simulink library "lib_transmission2"  (Simulink 4.1.1)
values from neighbouring files (symbols this model uses):
  logFlag = 1    [advSACompMaskInit.m]    (also in advSACompMaskInitR13.m)
undefined symbols (not defined in the file or in its folder): cyc_mph, fc_map_spd, fc_max_trq, fc_spd_scale, fc_trq_scale, fd_inertia, fd_loss, fd_ratio, gb_dnshift_load, gb_dnshift_spd, gb_gear_number_lookup, gb_gears_num, gb_inertia, gb_loss_const, gb_loss_input_spd_coeff, gb_loss_input_trq_coeff, gb_loss_output_spd_coeff, gb_loss_output_trq_coeff, gb_map_spd_out, gb_map_trq_in, gb_map_trq_out, gb_num_init, gb_ratio, gb_shift_delay, gb_spd_scale, gb_trq_scale, gb_upshift_load, gb_upshift_spd, htc_inertia, htc_k_adv, htc_k_adv_coast, htc_lockup, htc_lockup_load, htc_lockup_spd, htc_lu_gear_range, htc_max_coast_tr, htc_min_coast_tr, htc_pump_loss_spd, htc_pump_loss_trq_lockup, htc_pump_loss_trq_unlock, htc_sr, htc_sr_coast, htc_tr, htc_tr_coast, htc_unlock_spd, mc_map_spd, mc_max_trq, mc_overtrq_factor, mc_spd_scale, mc_trq_scale, tc_loss, tc_mc_to_fc_ratio, tx_eff_map, tx_map_spd, tx_map_trq, tx_pg_r, tx_pg_s, tx_speed_dep, vc_clutch_bool, vc_idle_spd ... (+2)
libraries: lib_controls x1, lib_etc x1, lib_controls2 x1, lib_transmission x1
(part 2 of 17)

== system lib_transmission2/SubLibraries/loss (Nm) old methodology ==
  note: Loss torque applied at input side is a function of
      |  output speed, output torque, and gear number.
      | There is no loss if the gears are not turning.
  "output torque and speed (Nm), (rad/s)" : Inport  Port=1  LatchInput=off
  gear ratio : Inport  Port=2  LatchInput=off
  Abs : Abs  SaturateOnIntegerOverflow=on
  Block NOTES : Subsystem
      settings: RTWFcnNameOpts=Auto  RTWFileNameOpts=Auto
      mask Display: disp('Block\nNOTES')
  Constant : Constant  Orientation=up  Value=eps
  Constant1 : Constant  Value=gb_loss_input_spd_coeff/gb_spd_scale
  Constant2 : Constant  Value=gb_loss_input_trq_coeff/gb_trq_scale
  Constant3 : Constant  Value=gb_loss_output_spd_coeff/gb_spd_scale
  Constant4 : Constant  Value=gb_loss_output_trq_coeff/gb_trq_scale
  Constant5 : Constant  Orientation=up  Value=gb_loss_const
  Constant6 : Constant  Value=gb_loss_output_pwr_coeff/gb_spd_scale/gb_trq_scale
  Constant7 : Constant  Orientation=up  Value=0
  Demux : Demux  Outputs=2  BusSelectionMode=off
  Product : Product  Inputs=2  Multiplication=Element-wise(.*)  SaturateOnIntegerOverflow=on
  Product1 : Product  Inputs=/*  Multiplication=Element-wise(.*)  SaturateOnIntegerOverflow=on
  Product2 : Product  Inputs=2  Multiplication=Element-wise(.*)  SaturateOnIntegerOverflow=on
  Product3 : Product  Inputs=2  Multiplication=Element-wise(.*)  SaturateOnIntegerOverflow=on
  Product4 : Product  Inputs=3  Multiplication=Element-wise(.*)  SaturateOnIntegerOverflow=on
  Relational Operator : RelationalOperator  Operator=>
  Saturation : Saturate  UpperLimit=inf  LowerLimit=0  LinearizeAsGain=on
  Sum : Sum  Inputs=++  SaturateOnIntegerOverflow=on
  Sum1 : Sum  Inputs=++  SaturateOnIntegerOverflow=on
  Sum2 : Sum  Inputs=++++  SaturateOnIntegerOverflow=on
  Sum3 : Sum  Orientation=up  Inputs=++  SaturateOnIntegerOverflow=on
  Switch : Switch  Threshold=eps
  loss torque : Product  Inputs=*//  Multiplication=Element-wise(.*)  SaturateOnIntegerOverflow=on
  loss torque at input shaft (Nm) : Outport  Port=1  InitialOutput=0
  wires:
  Abs/1 -> Product2/1, Product4/1
  Demux/1 -> Abs/1
  Relational Operator/1 -> Switch/2
  Constant/1 -> Relational Operator/2, Sum3/2
  Constant7/1 -> Switch/3
  Product3/1 -> Sum2/3
  Product2/1 -> Sum2/1
  "output torque and speed (Nm), (rad/s)"/1 -> Demux/1
  Constant1/1 -> Product/2
  Product/1 -> Sum1/2
  Sum/1 -> Product2/2
  Sum1/1 -> Product3/2
  Constant5/1 -> Sum2/4
  gear ratio/1 -> Product1/1, Product/1, loss torque/3
  Constant2/1 -> Product1/2
  Product1/1 -> Sum/2
  Constant4/1 -> Sum/1
  Constant3/1 -> Sum1/1
  Constant6/1 -> Product4/2
  Product4/1 -> Sum2/2
  Switch/1 -> loss torque at input shaft (Nm)/1
  Sum2/1 -> loss torque/1
  Demux/2 -> Product3/1, Product4/3, Relational Operator/1, Sum3/1
  loss torque/1 -> Saturation/1
  Saturation/1 -> Switch/1
  Sum3/1 -> loss torque/2

== system lib_transmission2/SubLibraries/notes on  3D discrete lookup table ==
  note: performs a "2D" lookup
      | for the specified
      | z height of the 3D lookup matrix
      | (i.e., no interpolation on z, only discrete)
  note: created 5 July 2001 mpo
      | Revision history:
      | ...
  note: 3 inputs:
      | (1) X lookup
      | (2) Y lookup
      | (3) discrete Z value (integer)
      |
      | 1 output:
      | (1) looked up value
  note: 3 masked inputs:
      | (1) array of X values in table
      | (2) array of Y values in table
      | (3) 3D lookup table (i.e., 2D tables for several Z values)

== system lib_transmission2/SubLibraries/notes on  loss (Nm) ==
  note: 4 masked inputs:
      | (1) map of efficiencies by spd and trq and gear number (discrete)
      | (2) array of trq values in efficiency map lookup table
      | (3) array of spd values in efficiency map lookup table
      | (4) the ratios in the gear box
  note: 2 inputs:
      | (1) trq and spd at output (wheel side)
      | of Transmission (muxxed)
      | (2) current gear ratio
      |
      | 1 output:
      | (1) trq loss at input (engine side) of
      | transmission
  note: created 5 July 2001 mpo
      | Revision history:
      | ...
  note: Calculates the torque loss due to
      | transmission inefficiencies
      | (torque lost at input to transmission)
  note: note: tx_map_spd and tx_map_trq
      |  are output (wheelside) values
  note: data needs:
      | tx_map_spd
      | tx_map_trq
      | tx_eff_map
      | gb_ratio

== system lib_transmission2/clutch <cl>/clutch model and interface ==
  note: Interface
  note: Model
  T & w output requested : Inport  Port=1  LatchInput=off
  T & w input achieved : Inport  Port=2  LatchInput=off
  control : Inport  Port=3  LatchInput=off
  Bus Creator : BusCreator  Inputs=2
  Demux2 : Demux  Outputs=3  BusSelectionMode=off
  Goto Tag Visibility : GotoTagVisibility  GotoTag=clutch_state
  Goto Tag Visibility1 : GotoTagVisibility  GotoTag=T_cl_out
  Goto Tag Visibility2 : GotoTagVisibility  GotoTag=w_cl_out
  Goto Tag Visibility3 : GotoTagVisibility  GotoTag=launch_speed
  Goto Tag Visibility4 : GotoTagVisibility  GotoTag=launch_flag
  clutch model : Subsystem
      settings: RTWFcnNameOpts=Auto  RTWFileNameOpts=Auto
  signal annotator : Subsystem
      settings: RTWFcnNameOpts=Auto  RTWFileNameOpts=Auto
  required out : Outport  Port=1
  Out1 : Outport  Port=2
  Out2 : Outport  Port=3
  sensors : Outport  Port=4
  tag scope: clutch_state=scoped, launch_flag=scoped, launch_speed=scoped
  wires:
  control/1 -> Demux2/1
  Demux2/1 -> [clutch_state]
  Demux2/2 -> [launch_speed]
  Demux2/3 -> [launch_flag]
  [T_cl_out] -> Bus Creator/1  "T_cl_out"
  [w_cl_out] -> Bus Creator/2  "w_cl_out"
  T & w output requested/1 -> clutch model/1(T & w output requested), signal annotator/1(In1)
  clutch model/1(T & w input request) -> Out1/1
  T & w input achieved/1 -> clutch model/2(T & w input achieved)
  clutch model/2(T & w output achieved) -> Out2/1
  Bus Creator/1 -> sensors/1
  signal annotator/1(Out1) -> required out/1

== system lib_transmission2/final drive <fd>/Block NOTES ==
  note: This final drive model includes loss data, rotational inertia, and a gear reduction.
  note: The loss torque is zero when the gears are not turning,
      | and is applied at the input side of the gear reduction.
  note: The inertia torque is the input torque required to accelerate the
      | final drive's inertia as measured on the input side.

== system lib_transmission2/final drive <fd>/help ==

== system lib_transmission2/final drive <fd>/model&interface ==
  note: Interface
  note: Model
  T & w output request : Inport  Port=1  LatchInput=off
  T & w input achieved : Inport  Port=2  LatchInput=off
  control : Inport  Port=3  LatchInput=off
  Ground : Ground
  Terminator : Terminator
  model : Subsystem
      settings: RTWFcnNameOpts=Auto  RTWFileNameOpts=Auto
  signal annotator : Subsystem
      settings: RTWFcnNameOpts=Auto  RTWFileNameOpts=Auto
  out request : Outport  Port=1  InitialOutput=0
  T & w input request : Outport  Port=2  InitialOutput=0
  T & w output achieved : Outport  Port=3  InitialOutput=0
  sensors : Outport  Port=4  InitialOutput=0
  wires:
  model/1("torque and speed req'd at input side of final drive (Nm), (rad/s)") -> T & w input request/1
  T & w output request/1 -> model/1("torque and speed req'd at output side of final drive (Nm), (rad/s)"), signal annotator/1(In1)
  T & w input achieved/1 -> model/2("torque and speed avail. at input side of final drive (Nm), (rad/s)")
  model/2("torque and speed avail. at output side of final drive (Nm), (rad/s)") -> T & w output achieved/1
  Ground/1 -> sensors/1
  control/1 -> Terminator/1
  signal annotator/1(Out1) -> out request/1

== system lib_transmission2/gearbox <gb>/Block NOTES ==
  note: This gearbox model includes loss data, rotational inertia, and a gear reduction.
  note: The loss torque is zero when the gears are not turning,
      | and is applied at the input side of the gear reduction.
  note: The inertia torque is the input torque required to accelerate the
      | final drive's inertia as measured on the input side.
  note: Available output torque is estimated assuming that the gearbox efficiency for theavailable input
      | torque andspeed is the same as the gearbox efficiency for the REQUESTED input torque.
  note: This is a good assumption, at least for the VW 4-speed manual transaxle of SAE 820741.
      | In the VW transaxle, efficiency is fairly independent of torque and speed at high torques.

== system lib_transmission2/gearbox <gb>/gearbox model & interface ==
  note: Model
  note: Interface
  trq and spd output request : Inport  Port=1  LatchInput=off
  trq and spd input achieved : Inport  Port=2  LatchInput=off
  controls : Inport  Port=3  LatchInput=off
  Bus Creator : BusCreator  Inputs=6
  Demux2 : Demux  Outputs=3  BusSelectionMode=off
  Goto Tag Visibility : GotoTagVisibility  GotoTag=gear_number
  Goto Tag Visibility1 : GotoTagVisibility  GotoTag=gb_spd_in_a
  Goto Tag Visibility2 : GotoTagVisibility  GotoTag=gear_ratio
  Goto Tag Visibility3 : GotoTagVisibility  GotoTag=shifting
  Goto Tag Visibility4 : GotoTagVisibility  GotoTag=T_gb_out
  Goto Tag Visibility5 : GotoTagVisibility  GotoTag=w_gb_out
  Goto Tag Visibility6 : GotoTagVisibility  GotoTag=eta_gb
  Goto Tag Visibility7 : GotoTagVisibility  GotoTag=gb_trq_out_a
  Goto Tag Visibility8 : GotoTagVisibility  GotoTag=gb_spd_out_a
  gearbox model : Subsystem
      settings: RTWFcnNameOpts=Auto  RTWFileNameOpts=Auto
  signal annotator : Subsystem
      settings: RTWFcnNameOpts=Auto  RTWFileNameOpts=Auto
  requested output : Outport  Port=1
  trq and spd input request : Outport  Port=2
  trq and spd output achieved : Outport  Port=3
  sensors : Outport  Port=4
  tag scope: gear_number=scoped, gear_ratio=scoped, shifting=scoped
  wires:
  [gb_spd_out_a] -> Bus Creator/6  "gb_spd_out_a"
  [gb_spd_in_a] -> Bus Creator/1  "gb_spd_in_a"
  [T_gb_out] -> Bus Creator/2  "T_gb_out"
  [w_gb_out] -> Bus Creator/3  "w_gb_out"
  [eta_gb] -> Bus Creator/4  "eta_gb"
  Bus Creator/1 -> sensors/1
  controls/1 -> Demux2/1
  Demux2/1 -> [gear_ratio]
  Demux2/2 -> [shifting]
  Demux2/3 -> [gear_number]
  trq and spd output request/1 -> gearbox model/1("torque and speed req'd at output side of gearbox (Nm), (rad/s)"), signal annotator/1(In1)
  gearbox model/1("torque and speed req'd at input side of gearbox (Nm), (rad/s)") -> trq and spd input request/1
  trq and spd input achieved/1 -> gearbox model/2("torque and speed avail. at input side of gearbox (Nm), (rad/s)")
  gearbox model/2("torque and speed avail. at output side of gearbox (Nm), (rad/s)") -> trq and spd output achieved/1
  signal annotator/1(Out1) -> requested output/1
  [gb_trq_out_a] -> Bus Creator/5  "gb_trq_out_a"

== system lib_transmission2/gearbox <gb>/help ==

== system lib_transmission2/gearbox <gb> CVT/Block NOTES ==
  note: This gearbox model includes loss data, rotational inertia, and a gear reduction.
  note: The loss torque is zero when the gears are not turning,
      | and is applied at the input side of the gear reduction.
  note: The inertia torque is the input torque required to accelerate the
      | final drive's inertia as measured on the input side.
  note: Available output torque is estimated assuming that the gearbox efficiency for theavailable input
      | torque andspeed is the same as the gearbox efficiency for the REQUESTED input torque.
  note: This is a good assumption, at least for the VW 4-speed manual transaxle of SAE 820741.
      | In the VW transaxle, efficiency is fairly independent of torque and speed at high torques.

== system lib_transmission2/gearbox <gb> CVT/CVT model & interface ==
  note: Model
  note: Interface
  trq and spd output request : Inport  Port=1  LatchInput=off
  trq and spd input achieved : Inport  Port=2  LatchInput=off
  controls : Inport  Port=3  LatchInput=off
  Bus Creator : BusCreator  Inputs=3
  CVT gearbox  <gb> : Subsystem
      settings: RTWFcnNameOpts=Auto  RTWFileNameOpts=Auto
  Demux2 : Demux  Outputs=1  BusSelectionMode=off
  Goto Tag Visibility2 : GotoTagVisibility  GotoTag=gear_ratio
  Goto Tag Visibility4 : GotoTagVisibility  GotoTag=T_gb_out
  Goto Tag Visibility5 : GotoTagVisibility  GotoTag=w_gb_out
  Goto Tag Visibility6 : GotoTagVisibility  GotoTag=eta_gb
  signal annotator : Subsystem
      settings: RTWFcnNameOpts=Auto  RTWFileNameOpts=Auto
  requested output : Outport  Port=1
  trq and spd input request : Outport  Port=2
  trq and spd output achieved : Outport  Port=3
  sensors : Outport  Port=4
  tag scope: gear_ratio=scoped
  wires:
  Bus Creator/1 -> sensors/1
  controls/1 -> Demux2/1
  Demux2/1 -> [gear_ratio]
  trq and spd output request/1 -> signal annotator/1(In1), CVT gearbox  <gb>/1("torque and speed req'd at output side of cvt (Nm), (rad/s)")
  CVT gearbox  <gb>/1("torque and speed req'd at input side of cvt (Nm), (rad/s)") -> trq and spd input request/1
  trq and spd input achieved/1 -> CVT gearbox  <gb>/2("torque and speed avail. at input side of cvt (Nm), (rad/s)")
  CVT gearbox  <gb>/2("torque and speed avail. at output side of cvt (Nm), (rad/s)") -> trq and spd output achieved/1
  signal annotator/1(Out1) -> requested output/1
  [T_gb_out] -> Bus Creator/1  "T_gb_out"
  [w_gb_out] -> Bus Creator/2  "w_gb_out"
  [eta_gb] -> Bus Creator/3  "eta_gb"

== system lib_transmission2/gearbox <gb> CVT/help ==

== system lib_transmission2/gearbox <gb> old/Block NOTES ==
  note: This gearbox model includes loss data, rotational inertia, and a gear reduction.
  note: The loss torque is zero when the gears are not turning,
      | and is applied at the input side of the gear reduction.
  note: The inertia torque is the input torque required to accelerate the
      | final drive's inertia as measured on the input side.
  note: Available output torque is estimated assuming that the gearbox efficiency for theavailable input
      | torque andspeed is the same as the gearbox efficiency for the REQUESTED input torque.
  note: This is a good assumption, at least for the VW 4-speed manual transaxle of SAE 820741.
      | In the VW transaxle, efficiency is fairly independent of torque and speed at high torques.

== system lib_transmission2/gearbox <gb> old/gearbox model & interface ==
  note: Model
  note: Interface
  trq and spd output request : Inport  Port=1  LatchInput=off
  trq and spd input achieved : Inport  Port=2  LatchInput=off
  controls : Inport  Port=3  LatchInput=off
  Bus Creator : BusCreator  Inputs=5
  Demux2 : Demux  Outputs=3  BusSelectionMode=off
  Goto Tag Visibility : GotoTagVisibility  GotoTag=gear_number
  Goto Tag Visibility1 : GotoTagVisibility  GotoTag=gb_spd_in_a
  Goto Tag Visibility2 : GotoTagVisibility  GotoTag=gear_ratio
  Goto Tag Visibility3 : GotoTagVisibility  GotoTag=shifting
  Goto Tag Visibility4 : GotoTagVisibility  GotoTag=T_gb_out
  Goto Tag Visibility5 : GotoTagVisibility  GotoTag=w_gb_out
  Goto Tag Visibility6 : GotoTagVisibility  GotoTag=eta_gb
  Goto Tag Visibility7 : GotoTagVisibility  GotoTag=gb_trq_out_a
  gearbox model : Subsystem
      settings: RTWFcnNameOpts=Auto  RTWFileNameOpts=Auto
  signal annotator : Subsystem
      settings: RTWFcnNameOpts=Auto  RTWFileNameOpts=Auto
  requested output : Outport  Port=1
  trq and spd input request : Outport  Port=2
  trq and spd output achieved : Outport  Port=3
  sensors : Outport  Port=4
  tag scope: gear_number=scoped, gear_ratio=scoped, shifting=scoped
  wires:
  [gb_spd_in_a] -> Bus Creator/1  "gb_spd_in_a"
  [T_gb_out] -> Bus Creator/2  "T_gb_out"
  [w_gb_out] -> Bus Creator/3  "w_gb_out"
  [eta_gb] -> Bus Creator/4  "eta_gb"
  Bus Creator/1 -> sensors/1
  controls/1 -> Demux2/1
  Demux2/1 -> [gear_ratio]
  Demux2/2 -> [shifting]
  Demux2/3 -> [gear_number]
  trq and spd output request/1 -> gearbox model/1("torque and speed req'd at output side of gearbox (Nm), (rad/s)"), signal annotator/1(In1)
  gearbox model/1("torque and speed req'd at input side of gearbox (Nm), (rad/s)") -> trq and spd input request/1
  trq and spd input achieved/1 -> gearbox model/2("torque and speed avail. at input side of gearbox (Nm), (rad/s)")
  gearbox model/2("torque and speed avail. at output side of gearbox (Nm), (rad/s)") -> trq and spd output achieved/1
  signal annotator/1(Out1) -> requested output/1
  [gb_trq_out_a] -> Bus Creator/5  "gb_trq_out_a"

== system lib_transmission2/gearbox <gb> old/help ==

== system lib_transmission2/hydraulic torque converter <htc>/conventional HTC  and Interface ==
  note: Model
  note: Interface
  trq and spd output request : Inport  Port=1  LatchInput=off
  trq and spd input achieved : Inport  Port=2  LatchInput=off
  control : Inport  Port=3  LatchInput=off
  Bus Creator : BusCreator  Inputs=1
  Demux : Demux  Outputs=2  BusSelectionMode=off
  Goto Tag Visibility : GotoTagVisibility  GotoTag=shifting
  Goto Tag Visibility1 : GotoTagVisibility  GotoTag=htc_efficiency
  Goto Tag Visibility2 : GotoTagVisibility  GotoTag=locked_up
  htc model : Subsystem
      settings: RTWFcnNameOpts=Auto  RTWFileNameOpts=Auto
  signal annotator : Subsystem
      settings: RTWFcnNameOpts=Auto  RTWFileNameOpts=Auto
  requested output : Outport  Port=1  InitialOutput=0
  trq and spd input request : Outport  Port=2  InitialOutput=0
  trq and spd output achieved : Outport  Port=3  InitialOutput=0
  sensors : Outport  Port=4  InitialOutput=0
  tag scope: locked_up=scoped, shifting=scoped
  wires:
  trq and spd output request/1 -> htc model/1("req'd output trq and spd (Nm), (rad/s)"), signal annotator/1(In1)
  htc model/1("req'd input trq and spd (Nm), (rad/s)") -> trq and spd input request/1
  htc model/2("trq and spd available at output (Nm), (rad/s)") -> trq and spd output achieved/1
  trq and spd input achieved/1 -> htc model/2("trq and spd available at input (Nm), (rad/s)")
  signal annotator/1(Out1) -> requested output/1
  control/1 -> Demux/1
  Demux/1 -> [shifting]
  Demux/2 -> [locked_up]
  [htc_efficiency] -> Bus Creator/1  "htc_efficiency"
  Bus Creator/1 -> sensors/1

== system lib_transmission2/hydraulic torque converter <htc> HEV/HTC for parallel HEV and Interface ==
  note: Model
  note: Interface
  trq and spd output request : Inport  Port=1  LatchInput=off
  trq and spd input achieved : Inport  Port=2  LatchInput=off
  control : Inport  Port=3  LatchInput=off
  Demux : Demux  Outputs=2  BusSelectionMode=off
  Goto Tag Visibility : GotoTagVisibility  GotoTag=shifting
  Goto Tag Visibility2 : GotoTagVisibility  GotoTag=locked_up
  Ground : Ground
  model for parallel HEV : Subsystem
      settings: RTWFcnNameOpts=Auto  RTWFileNameOpts=Auto
  signal annotator : Subsystem
      settings: RTWFcnNameOpts=Auto  RTWFileNameOpts=Auto
  requested output : Outport  Port=1  InitialOutput=0
  trq and spd input request : Outport  Port=2  InitialOutput=0
  trq and spd output achieved : Outport  Port=3  InitialOutput=0
  sensors : Outport  Port=4  InitialOutput=0
  tag scope: locked_up=scoped, shifting=scoped
  wires:
  trq and spd output request/1 -> signal annotator/1(In1), model for parallel HEV/1("req'd output trq and spd (Nm), (rad/s)")
  model for parallel HEV/1("req'd input trq and spd (Nm), (rad/s)") -> trq and spd input request/1
  model for parallel HEV/2("trq and spd available at output (Nm), (rad/s)") -> trq and spd output achieved/1
  trq and spd input achieved/1 -> model for parallel HEV/2("trq and spd available at input (Nm), (rad/s)")
  signal annotator/1(Out1) -> requested output/1
  control/1 -> Demux/1
  Demux/1 -> [shifting]
  Demux/2 -> [locked_up]
  Ground/1 -> sensors/1

== system lib_transmission2/hydraulic torque converter <htc> with pump loss/conventional HTC  and Interface ==
  note: Model
  note: Interface
  trq and spd output request : Inport  Port=1  LatchInput=off
  trq and spd input achieved : Inport  Port=2  LatchInput=off
  control : Inport  Port=3  LatchInput=off
  Bus Creator : BusCreator  Inputs=1
  Demux : Demux  Outputs=2  BusSelectionMode=off
  Goto Tag Visibility : GotoTagVisibility  GotoTag=shifting
  Goto Tag Visibility1 : GotoTagVisibility  GotoTag=htc_efficiency
  Goto Tag Visibility2 : GotoTagVisibility  GotoTag=locked_up
  htc model : Subsystem
      settings: RTWFcnNameOpts=Auto  RTWFileNameOpts=Auto
  signal annotator : Subsystem
      settings: RTWFcnNameOpts=Auto  RTWFileNameOpts=Auto
  requested output : Outport  Port=1  InitialOutput=0
  trq and spd input request : Outport  Port=2  InitialOutput=0
  trq and spd output achieved : Outport  Port=3  InitialOutput=0
  sensors : Outport  Port=4  InitialOutput=0
  tag scope: locked_up=scoped, shifting=scoped
  wires:
  trq and spd output request/1 -> htc model/1("req'd output trq and spd (Nm), (rad/s)"), signal annotator/1(In1)
  htc model/1("req'd input trq and spd (Nm), (rad/s)") -> trq and spd input request/1
  htc model/2("trq and spd available at output (Nm), (rad/s)") -> trq and spd output achieved/1
  trq and spd input achieved/1 -> htc model/2("trq and spd available at input (Nm), (rad/s)")
  signal annotator/1(Out1) -> requested output/1
  control/1 -> Demux/1
  Demux/1 -> [shifting]
  Demux/2 -> [locked_up]
  [htc_efficiency] -> Bus Creator/1  "htc_efficiency"
  Bus Creator/1 -> sensors/1

== system lib_transmission2/torque coupler <tc>/tc model & interface ==
  note: Interface
  note: Model
  trq and spd output request : Inport  Port=1  LatchInput=off
  trq and spd avail. at main input : Inport  Port=2  LatchInput=off
  trq and spd avail. at motor input to tc : Inport  Port=3  LatchInput=off
  controls : Inport  Port=4  LatchInput=off
  Ground : Ground
  Terminator : Terminator
  signal annotator : Subsystem
      settings: RTWFcnNameOpts=Auto  RTWFileNameOpts=Auto
  tc model : Subsystem
      settings: RTWFcnNameOpts=Auto  RTWFileNameOpts=Auto
  requested output : Outport  Port=1
  trq and spd req'd at main input : Outport  Port=2  InitialOutput=0
  trq and spd req'd at motor input to torque coupler : Outport  Port=3  InitialOutput=0
  trq and spd avail. at output side of torque coupler : Outport  Port=4  InitialOutput=0
  sensors : Outport  Port=5
  wires:
  tc model/1("torque and speed req'd at main input to torque coupler (Nm), (rad/s)") -> trq and spd req'd at main input/1
  tc model/2("torque and speed req'd at motor input to torque coupler (Nm), (rad/s)") -> trq and spd req'd at motor input to torque coupler/1
  trq and spd avail. at main input/1 -> tc model/2("torque and speed avail. at main input (Nm), (rad/s)")
  tc model/3("torque and speed avail. at output side of torque coupler (Nm), (rad/s)") -> trq and spd avail. at output side of torque coupler/1
  trq and spd avail. at motor input to tc/1 -> tc model/3("torque and speed avail. at motor input to tc (Nm), (rad/s)")
  trq and spd output request/1 -> tc model/1("torque and speed req'd at output side of torque coupler (Nm), (rad/s)"), signal annotator/1(In1)
  signal annotator/1(Out1) -> requested output/1
  controls/1 -> Terminator/1
  Ground/1 -> sensors/1

== system lib_transmission2/torque coupler <tc> DIRECT SPLIT/tc direct split model & interface ==
  note: Interface
  note: Model
  trq and spd output request : Inport  Port=1  LatchInput=off
  trq and spd avail. at main input : Inport  Port=2  LatchInput=off
  trq and spd avail. at motor input to tc : Inport  Port=3  LatchInput=off
  control : Inport  Port=4  LatchInput=off
  Ground : Ground
  Terminator : Terminator
  signal annotator : Subsystem
      settings: RTWFcnNameOpts=Auto  RTWFileNameOpts=Auto
  tc direct split model : Subsystem
      settings: RTWFcnNameOpts=Auto  RTWFileNameOpts=Auto
  required output : Outport  Port=1
  trq and spd req'd at main input : Outport  Port=2
  trq and spd avail. at output side of torque coupler : Outport  Port=3
  sensors : Outport  Port=4
  wires:
  trq and spd output request/1 -> tc direct split model/1("torque and speed req'd at output side of torque coupler (Nm), (rad/s)"), signal annotator/1(In1)
  tc direct split model/1("torque and speed req'd at main input to torque coupler (Nm), (rad/s)") -> trq and spd req'd at main input/1
  trq and spd avail. at main input/1 -> tc direct split model/2("torque and speed avail. at main input (Nm), (rad/s)")
  tc direct split model/2("torque and speed avail. at output side of torque coupler (Nm), (rad/s)") -> trq and spd avail. at output side of torque coupler/1
  trq and spd avail. at motor input to tc/1 -> tc direct split model/3("torque and speed avail. at motor input to tc (Nm), (rad/s)")
  Ground/1 -> sensors/1
  control/1 -> Terminator/1
  signal annotator/1(Out1) -> required output/1

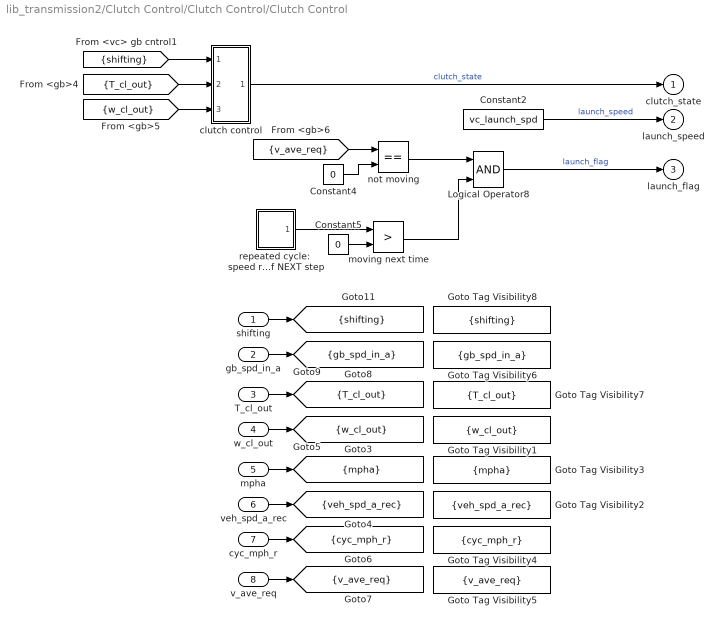
== system lib_transmission2/Clutch Control/Clutch Control/Clutch Control ==
  shifting : Inport  Port=1  LatchInput=off
  gb_spd_in_a : Inport  Port=2  LatchInput=off
  T_cl_out : Inport  Port=3  LatchInput=off
  w_cl_out : Inport  Port=4  LatchInput=off
  mpha : Inport  Port=5  LatchInput=off
  veh_spd_a_rec : Inport  Port=6  LatchInput=off
  cyc_mph_r : Inport  Port=7  LatchInput=off
  v_ave_req : Inport  Port=8  LatchInput=off
  Constant2 : Constant  Value=vc_launch_spd
  Constant4 : Constant  Value=0
  Constant5 : Constant  Value=0
  Goto Tag Visibility1 : GotoTagVisibility  GotoTag=w_cl_out
  Goto Tag Visibility2 : GotoTagVisibility  GotoTag=veh_spd_a_rec
  Goto Tag Visibility3 : GotoTagVisibility  GotoTag=mpha
  Goto Tag Visibility4 : GotoTagVisibility  GotoTag=cyc_mph_r
  Goto Tag Visibility5 : GotoTagVisibility  GotoTag=v_ave_req
  Goto Tag Visibility6 : GotoTagVisibility  GotoTag=gb_spd_in_a
  Goto Tag Visibility7 : GotoTagVisibility  GotoTag=T_cl_out
  Goto Tag Visibility8 : GotoTagVisibility  GotoTag=shifting
  Logical Operator8 : Logic  Operator=AND  Inputs=2
  clutch control : Subsystem
      settings: RTWFcnNameOpts=Auto  RTWFileNameOpts=Auto
  moving next time : RelationalOperator  Operator=>
  not moving : RelationalOperator  Operator===
  repeated cycle:  speed required at end of NEXT step : Subsystem  mask(Forward looking repeating table){t=cyc_mph(:,1), y=cyc_mph(:,2)}
      mask prompts: t "Time values:"; y "Output values:"
      mask help:
      | Forward looking repeating table.
      | Enter values of time and output for first cycle.
      mask init:
      | period = max(t);
      settings: RTWFcnNameOpts=Auto  RTWFileNameOpts=Auto
      mask Help: Repeats cycle given in table with a one time step forward offset. Time values should be monotonically increasing.
  clutch_state : Outport  Port=1  InitialOutput=0
  launch_speed : Outport  Port=2  InitialOutput=0
  launch_flag : Outport  Port=3  InitialOutput=0
  tag scope: T_cl_out=scoped, cyc_mph_r=scoped, gb_spd_in_a=scoped, mpha=scoped, shifting=scoped, v_ave_req=scoped, veh_spd_a_rec=scoped, w_cl_out=scoped
  wires:
  veh_spd_a_rec/1 -> [veh_spd_a_rec]
  T_cl_out/1 -> [T_cl_out]
  shifting/1 -> [shifting]
  gb_spd_in_a/1 -> [gb_spd_in_a]
  v_ave_req/1 -> [v_ave_req]
  cyc_mph_r/1 -> [cyc_mph_r]
  mpha/1 -> [mpha]
  w_cl_out/1 -> [w_cl_out]
  Constant2/1 -> launch_speed/1  "launch_speed"
  not moving/1 -> Logical Operator8/1
  Logical Operator8/1 -> launch_flag/1  "launch_flag"
  Constant4/1 -> not moving/2
  [v_ave_req] -> not moving/1
  repeated cycle:  speed required at end of NEXT step/1(out_1) -> moving next time/1
  Constant5/1 -> moving next time/2
  moving next time/1 -> Logical Operator8/2
  clutch control/1(clutch state) -> clutch_state/1  "clutch_state"
  [w_cl_out] -> clutch control/3(gb_spd_in_r)
  [T_cl_out] -> clutch control/2(gb_trq_in_r)
  [shifting] -> clutch control/1(shifting)

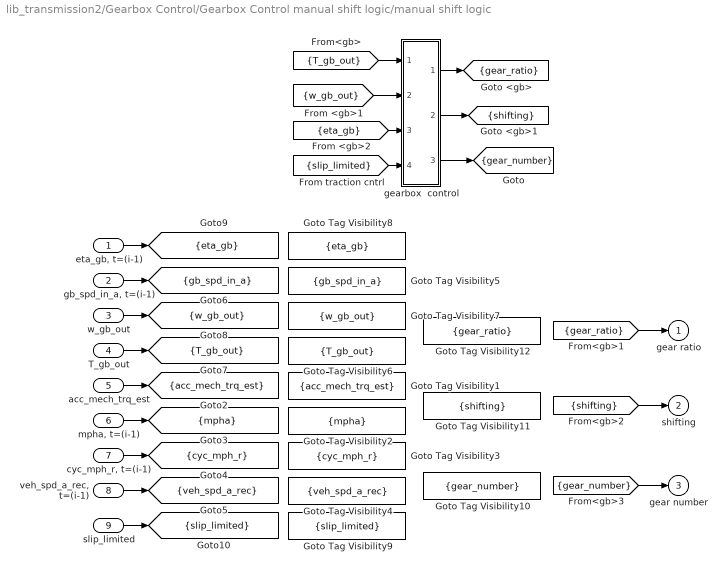
== system lib_transmission2/Gearbox Control/Gearbox Control manual shift logic/manual shift logic ==
  "eta_gb, t=(i-1)" : Inport  Port=1  LatchInput=off
  "gb_spd_in_a, t=(i-1)" : Inport  Port=2  LatchInput=off
  w_gb_out : Inport  Port=3  LatchInput=off
  T_gb_out : Inport  Port=4  LatchInput=off
  acc_mech_trq_est : Inport  Port=5  LatchInput=off
  "mpha, t=(i-1)" : Inport  Port=6  LatchInput=off
  "cyc_mph_r, t=(i-1)" : Inport  Port=7  LatchInput=off
  "veh_spd_a_rec, t=(i-1)" : Inport  Port=8  LatchInput=off
  slip_limited : Inport  Port=9  LatchInput=off
  Goto Tag Visibility1 : GotoTagVisibility  GotoTag=acc_mech_trq_est
  Goto Tag Visibility10 : GotoTagVisibility  GotoTag=gear_number
  Goto Tag Visibility11 : GotoTagVisibility  GotoTag=shifting
  Goto Tag Visibility12 : GotoTagVisibility  GotoTag=gear_ratio
  Goto Tag Visibility2 : GotoTagVisibility  GotoTag=mpha
  Goto Tag Visibility3 : GotoTagVisibility  GotoTag=cyc_mph_r
  Goto Tag Visibility4 : GotoTagVisibility  GotoTag=veh_spd_a_rec
  Goto Tag Visibility5 : GotoTagVisibility  GotoTag=gb_spd_in_a
  Goto Tag Visibility6 : GotoTagVisibility  GotoTag=T_gb_out
  Goto Tag Visibility7 : GotoTagVisibility  GotoTag=w_gb_out
  Goto Tag Visibility8 : GotoTagVisibility  GotoTag=eta_gb
  Goto Tag Visibility9 : GotoTagVisibility  GotoTag=slip_limited
  gearbox  control : Subsystem
      settings: RTWFcnNameOpts=Auto  RTWFileNameOpts=Auto
  gear ratio : Outport  Port=1  InitialOutput=0
  shifting : Outport  Port=2  InitialOutput=0
  gear number : Outport  Port=3  InitialOutput=0
  tag scope: T_gb_out=scoped, acc_mech_trq_est=scoped, cyc_mph_r=scoped, eta_gb=scoped, gb_spd_in_a=scoped, gear_number=scoped, gear_ratio=scoped, mpha=scoped, shifting=scoped, slip_limited=scoped, veh_spd_a_rec=scoped, w_gb_out=scoped
  wires:
  T_gb_out/1 -> [T_gb_out]
  w_gb_out/1 -> [w_gb_out]
  "gb_spd_in_a, t=(i-1)"/1 -> [gb_spd_in_a]
  [gear_number] -> gear number/1
  [shifting] -> shifting/1
  [gear_ratio] -> gear ratio/1
  gearbox  control/3(gear number) -> [gear_number]
  gearbox  control/2(shifting) -> [shifting]
  gearbox  control/1(gear ratio2) -> [gear_ratio]
  slip_limited/1 -> [slip_limited]
  "eta_gb, t=(i-1)"/1 -> [eta_gb]
  "veh_spd_a_rec, t=(i-1)"/1 -> [veh_spd_a_rec]
  "cyc_mph_r, t=(i-1)"/1 -> [cyc_mph_r]
  "mpha, t=(i-1)"/1 -> [mpha]
  acc_mech_trq_est/1 -> [acc_mech_trq_est]
  [slip_limited] -> gearbox  control/4(tires are at traction limit)
  [eta_gb] -> gearbox  control/3(prev. Pout/Pin)
  [w_gb_out] -> gearbox  control/2(gb_spd_out_r)
  [T_gb_out] -> gearbox  control/1(gb_trq_out_r)

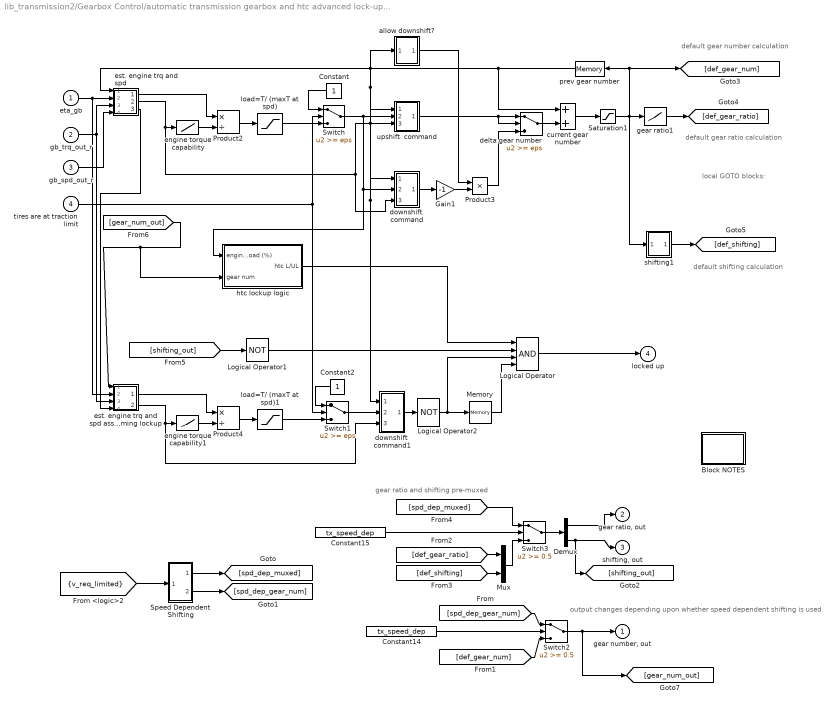
== system lib_transmission2/Gearbox Control/automatic transmission gearbox and htc advanced lock-up logic for htc shift logic for gearbox/gearbox control for use w/ AT ==
  note: output changes depending
      | upon whether speed
      | dependent shifting is used
  note: gear ratio and shifting pre-muxed
  note: local GOTO blocks:
  note: default gear ratio
      | calculation
  note: default shifting
      | calculation
  note: default gear number
      | calculation
  eta_gb : Inport  Port=1  LatchInput=off
  gb_trq_out_r : Inport  Port=2  LatchInput=off
  gb_spd_out_r : Inport  Port=3  LatchInput=off
  tires are at traction limit : Inport  Port=4  LatchInput=off
  Block NOTES : Subsystem
      settings: RTWFcnNameOpts=Auto  RTWFileNameOpts=Auto
      mask Display: disp('Block\nNOTES')
  Constant : Constant  Orientation=left  Value=1
  Constant14 : Constant  Value=tx_speed_dep
  Constant15 : Constant  Value=tx_speed_dep
  Constant2 : Constant  Orientation=left  Value=1
  Demux : Demux  Outputs=2  BusSelectionMode=off
  Gain1 : Gain  Gain=-1  Multiplication=Element-wise(K.*u)  SaturateOnIntegerOverflow=on
  Logical Operator : Logic  Operator=AND  Inputs=4
  Logical Operator1 : Logic  Operator=NOT  Inputs=1
  Logical Operator2 : Logic  Operator=NOT  Inputs=1
  Memory : Memory  X0=0  InheritSampleTime=off
      settings: RTWStateStorageClass=Auto
  Mux : Mux  Inputs=2
  Product2 : Product  Inputs=*/  Multiplication=Element-wise(.*)  SaturateOnIntegerOverflow=on
  Product3 : Product  Inputs=2  Multiplication=Element-wise(.*)  SaturateOnIntegerOverflow=on
  Product4 : Product  Inputs=*/  Multiplication=Element-wise(.*)  SaturateOnIntegerOverflow=on
  Saturation1 : Saturate  UpperLimit=gb_gears_num  LowerLimit=1  LinearizeAsGain=on
  Speed Dependent Shifting : Subsystem  AncestorBlock=lib_controls/SubSystem/Speed Dependent Shifting
      settings: RTWFcnNameOpts=Auto  RTWFileNameOpts=Auto
  Switch : Switch  Threshold=eps
  Switch1 : Switch  Threshold=eps
  Switch2 : Switch  Threshold=0.5
  Switch3 : Switch  Threshold=0.5
  allow downshift? : Subsystem
      settings: RTWFcnNameOpts=Auto  RTWFileNameOpts=Auto
  current gear number : Sum  Inputs=++  SaturateOnIntegerOverflow=on
  delta gear number : Switch  Threshold=eps
  downshift  command : Subsystem
      settings: RTWFcnNameOpts=Auto  RTWFileNameOpts=Auto
  downshift  command1 : Subsystem
      settings: RTWFcnNameOpts=Auto  RTWFileNameOpts=Auto
  engine torque capability : Lookup  InputValues=fc_map_spd*fc_spd_scale  OutputValues=fc_max_trq*fc_trq_scale+eps
  engine torque capability1 : Lookup  InputValues=fc_map_spd*fc_spd_scale  OutputValues=fc_max_trq*fc_trq_scale+eps
  est. engine trq and spd : Subsystem
      settings: RTWFcnNameOpts=Auto  RTWFileNameOpts=Auto
  est. engine trq and spd assuming lockup : Subsystem
      settings: RTWFcnNameOpts=Auto  RTWFileNameOpts=Auto
  gear ratio1 : Lookup  InputValues=[1:length(gb_ratio)]  OutputValues=gb_ratio
  htc lockup logic : Subsystem
      settings: RTWFcnNameOpts=Auto  RTWFileNameOpts=Auto
  load=T/ (maxT at spd) : Saturate  UpperLimit=1  LowerLimit=-1  LinearizeAsGain=on
  load=T/ (maxT at spd)1 : Saturate  UpperLimit=1  LowerLimit=-1  LinearizeAsGain=on
  prev gear number : Memory  Orientation=left  X0=gb_num_init  InheritSampleTime=off
      settings: RTWStateStorageClass=Auto
  shifting1 : Subsystem
      settings: RTWFcnNameOpts=Auto  RTWFileNameOpts=Auto
  upshift  command : Subsystem
      settings: RTWFcnNameOpts=Auto  RTWFileNameOpts=Auto
  "gear number, out" : Outport  Port=1  InitialOutput=0
  "gear ratio, out" : Outport  Port=2  InitialOutput=0
  "shifting, out" : Outport  Port=3  InitialOutput=0
  locked up : Outport  Port=4  InitialOutput=0
  wires:
  Demux/1 -> "gear ratio, out"/1
  [gear_num_out] -> est. engine trq and spd assuming lockup/1(new gear number), htc lockup logic/2(gear num)
  [shifting_out] -> Logical Operator1/1
  shifting1/1(out_1) -> [def_shifting]
  Switch2/1 -> [gear_num_out], "gear number, out"/1
  Demux/2 -> [shifting_out], "shifting, out"/1
  Speed Dependent Shifting/2(gear number) -> [spd_dep_gear_num]
  Speed Dependent Shifting/1(gear ratio and shifting) -> [spd_dep_muxed]
  [v_req_limited] -> Speed Dependent Shifting/1("velocity required (limited) ")
  [def_gear_num] -> Switch2/3
  [spd_dep_gear_num] -> Switch2/1
  Constant14/1 -> Switch2/2
  Switch3/1 -> Demux/1
  [def_shifting] -> Mux/2
  [def_gear_ratio] -> Mux/1
  Mux/1 -> Switch3/3
  [spd_dep_muxed] -> Switch3/1
  Constant15/1 -> Switch3/2
  prev gear number/1 -> est. engine trq and spd/1(prev gear number), allow downshift?/1(prev gearnum), downshift  command1/1(prev gear number), downshift  command/1(prev gear number), upshift  command/1(prev gear number), current gear number/1
  current gear number/1 -> Saturation1/1
  delta gear number/1 -> current gear number/2
  gear ratio1/1 -> [def_gear_ratio]
  downshift  command1/1(command) -> Logical Operator2/1
  load=T/ (maxT at spd)1/1 -> Switch1/3
  Memory/1 -> Logical Operator/4
  Switch1/1 -> downshift  command1/2(engine load)
  Logical Operator/1 -> locked up/1
  Gain1/1 -> Product3/2
  upshift  command/1(command) -> delta gear number/1, delta gear number/2
  Switch/1 -> upshift  command/2(engine load), downshift  command/2(engine load), htc lockup logic/1(engine load (%))
  Logical Operator2/1 -> Memory/1, Logical Operator/3
  est. engine trq and spd assuming lockup/2(est eng spd (rad/s)) -> downshift  command1/3(engine speed), engine torque capability1/1
  est. engine trq and spd/3(gb_spd_in_est (rad/s)1) -> est. engine trq and spd assuming lockup/4(gb_spd_in_est)
  tires are at traction limit/1 -> Switch/2, Switch1/2
  gb_trq_out_r/1 -> est. engine trq and spd assuming lockup/3(gb_trq_out_r), est. engine trq and spd/3(gb_trq_out_r)
  eta_gb/1 -> est. engine trq and spd assuming lockup/2(" prev eta_gb"), est. engine trq and spd/2(" prev eta_gb")
  est. engine trq and spd assuming lockup/1(est eng trq (Nm)) -> Product4/1
  engine torque capability1/1 -> Product4/2
  Product4/1 -> load=T/ (maxT at spd)1/1
  Constant2/1 -> Switch1/1
  htc lockup logic/1(htc L/UL) -> Logical Operator/1
  Logical Operator1/1 -> Logical Operator/2
  downshift  command/1(command) -> Gain1/1
  load=T/ (maxT at spd)/1 -> Switch/3
  est. engine trq and spd/1(est eng trq (Nm)) -> Product2/1
  engine torque capability/1 -> Product2/2
  Product3/1 -> delta gear number/3
  allow downshift?/1(allow shift) -> Product3/1
  Product2/1 -> load=T/ (maxT at spd)/1
  Constant/1 -> Switch/1
  Saturation1/1 -> shifting1/1(gear number), [def_gear_num], prev gear number/1, gear ratio1/1
  gb_spd_out_r/1 -> est. engine trq and spd/4(gb_spd_out_r)
  est. engine trq and spd/2(est eng spd (rad/s)) -> engine torque capability/1, upshift  command/3(engine speed), downshift  command/3(engine speed)

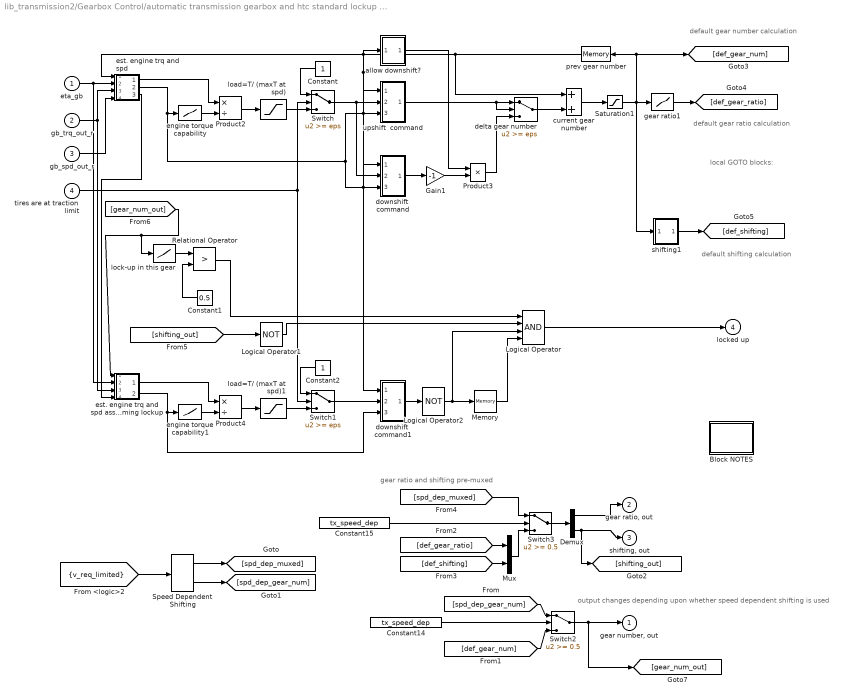
== system lib_transmission2/Gearbox Control/automatic transmission gearbox and htc standard lockup logic for htc shift logic for gearbox/gearbox control for use w/ AT ==
  note: default gear number
      | calculation
  note: default shifting
      | calculation
  note: default gear ratio
      | calculation
  note: local GOTO blocks:
  note: gear ratio and shifting pre-muxed
  note: output changes depending
      | upon whether speed
      | dependent shifting is used
  eta_gb : Inport  Port=1  LatchInput=off
  gb_trq_out_r : Inport  Port=2  LatchInput=off
  gb_spd_out_r : Inport  Port=3  LatchInput=off
  tires are at traction limit : Inport  Port=4  LatchInput=off
  Block NOTES : Subsystem
      settings: RTWFcnNameOpts=Auto  RTWFileNameOpts=Auto
      mask Display: disp('Block\nNOTES')
  Constant : Constant  Orientation=left  Value=1
  Constant1 : Constant  Orientation=left  Value=0.5
  Constant14 : Constant  Value=tx_speed_dep
  Constant15 : Constant  Value=tx_speed_dep
  Constant2 : Constant  Orientation=left  Value=1
  Demux : Demux  Outputs=2  BusSelectionMode=off
  Gain1 : Gain  Gain=-1  Multiplication=Element-wise(K.*u)  SaturateOnIntegerOverflow=on
  Logical Operator : Logic  Operator=AND  Inputs=4
  Logical Operator1 : Logic  Operator=NOT  Inputs=1
  Logical Operator2 : Logic  Operator=NOT  Inputs=1
  Memory : Memory  X0=0  InheritSampleTime=off
      settings: RTWStateStorageClass=Auto
  Mux : Mux  Inputs=2
  Product2 : Product  Inputs=*/  Multiplication=Element-wise(.*)  SaturateOnIntegerOverflow=on
  Product3 : Product  Inputs=2  Multiplication=Element-wise(.*)  SaturateOnIntegerOverflow=on
  Product4 : Product  Inputs=*/  Multiplication=Element-wise(.*)  SaturateOnIntegerOverflow=on
  Relational Operator : RelationalOperator  Operator=>
  Saturation1 : Saturate  UpperLimit=gb_gears_num  LowerLimit=1  LinearizeAsGain=on
  Speed Dependent Shifting : lib_controls/SubSystem/Speed Dependent Shifting
      settings: RTWFcnNameOpts=Auto  RTWFileNameOpts=Auto
  Switch : Switch  Threshold=eps
  Switch1 : Switch  Threshold=eps
  Switch2 : Switch  Threshold=0.5
  Switch3 : Switch  Threshold=0.5
  allow downshift? : Subsystem
      settings: RTWFcnNameOpts=Auto  RTWFileNameOpts=Auto
  current gear number : Sum  Inputs=++  SaturateOnIntegerOverflow=on
  delta gear number : Switch  Threshold=eps
  downshift  command : Subsystem
      settings: RTWFcnNameOpts=Auto  RTWFileNameOpts=Auto
  downshift  command1 : Subsystem
      settings: RTWFcnNameOpts=Auto  RTWFileNameOpts=Auto
  engine torque capability : Lookup  InputValues=fc_map_spd*fc_spd_scale  OutputValues=fc_max_trq*fc_trq_scale+eps
  engine torque capability1 : Lookup  InputValues=fc_map_spd*fc_spd_scale  OutputValues=fc_max_trq*fc_trq_scale+eps
  est. engine trq and spd : Subsystem
      settings: RTWFcnNameOpts=Auto  RTWFileNameOpts=Auto
  est. engine trq and spd assuming lockup : Subsystem
      settings: RTWFcnNameOpts=Auto  RTWFileNameOpts=Auto
  gear ratio1 : Lookup  InputValues=[1:length(gb_ratio)]  OutputValues=gb_ratio
  load=T/ (maxT at spd) : Saturate  UpperLimit=1  LowerLimit=-1  LinearizeAsGain=on
  load=T/ (maxT at spd)1 : Saturate  UpperLimit=1  LowerLimit=-1  LinearizeAsGain=on
  lock-up in this gear : Lookup  InputValues=[1:length(htc_lockup)]  OutputValues=htc_lockup
  prev gear number : Memory  Orientation=left  X0=gb_num_init  InheritSampleTime=off
      settings: RTWStateStorageClass=Auto
  shifting1 : Subsystem
      settings: RTWFcnNameOpts=Auto  RTWFileNameOpts=Auto
  upshift  command : Subsystem
      settings: RTWFcnNameOpts=Auto  RTWFileNameOpts=Auto
  "gear number, out" : Outport  Port=1  InitialOutput=0
  "gear ratio, out" : Outport  Port=2  InitialOutput=0
  "shifting, out" : Outport  Port=3  InitialOutput=0
  locked up : Outport  Port=4  InitialOutput=0
  wires:
  est. engine trq and spd/2(est eng spd (rad/s)) -> downshift  command/3(engine speed), upshift  command/3(engine speed), engine torque capability/1
  gb_spd_out_r/1 -> est. engine trq and spd/4(gb_spd_out_r)
  Saturation1/1 -> gear ratio1/1, prev gear number/1, [def_gear_num], shifting1/1(gear number)
  Constant/1 -> Switch/1
  Product2/1 -> load=T/ (maxT at spd)/1
  allow downshift?/1(allow shift) -> Product3/1
  Product3/1 -> delta gear number/3
  engine torque capability/1 -> Product2/2
  est. engine trq and spd/1(est eng trq (Nm)) -> Product2/1
  load=T/ (maxT at spd)/1 -> Switch/3
  downshift  command/1(command) -> Gain1/1
  Logical Operator1/1 -> Logical Operator/2
  Constant1/1 -> Relational Operator/2
  lock-up in this gear/1 -> Relational Operator/1
  Relational Operator/1 -> Logical Operator/1
  Constant2/1 -> Switch1/1
  Product4/1 -> load=T/ (maxT at spd)1/1
  engine torque capability1/1 -> Product4/2
  est. engine trq and spd assuming lockup/1(est eng trq (Nm)) -> Product4/1
  eta_gb/1 -> est. engine trq and spd/2(" prev eta_gb"), est. engine trq and spd assuming lockup/2(" prev eta_gb")
  gb_trq_out_r/1 -> est. engine trq and spd/3(gb_trq_out_r), est. engine trq and spd assuming lockup/3(gb_trq_out_r)
  tires are at traction limit/1 -> Switch1/2, Switch/2
  est. engine trq and spd/3(gb_spd_in_est (rad/s)) -> est. engine trq and spd assuming lockup/4(gb_spd_in_est)
  est. engine trq and spd assuming lockup/2(est eng spd (rad/s)) -> engine torque capability1/1, downshift  command1/3(engine speed)
  Logical Operator2/1 -> Logical Operator/3, Memory/1
  Switch/1 -> downshift  command/2(engine load), upshift  command/2(engine load)
  upshift  command/1(command) -> delta gear number/2, delta gear number/1
  Gain1/1 -> Product3/2
  Logical Operator/1 -> locked up/1
  Switch1/1 -> downshift  command1/2(engine load)
  Memory/1 -> Logical Operator/4
  load=T/ (maxT at spd)1/1 -> Switch1/3
  downshift  command1/1(command) -> Logical Operator2/1
  gear ratio1/1 -> [def_gear_ratio]
  delta gear number/1 -> current gear number/2
  current gear number/1 -> Saturation1/1
  prev gear number/1 -> current gear number/1, upshift  command/1(prev gear number), downshift  command/1(prev gear number), downshift  command1/1(prev gear number), allow downshift?/1(prev gearnum), est. engine trq and spd/1(prev gear number)
  Constant15/1 -> Switch3/2
  [spd_dep_muxed] -> Switch3/1
  Mux/1 -> Switch3/3
  [def_gear_ratio] -> Mux/1
  [def_shifting] -> Mux/2
  Switch3/1 -> Demux/1
  Constant14/1 -> Switch2/2
  [spd_dep_gear_num] -> Switch2/1
  [def_gear_num] -> Switch2/3
  [v_req_limited] -> Speed Dependent Shifting/1
  Speed Dependent Shifting/1 -> [spd_dep_muxed]
  Speed Dependent Shifting/2 -> [spd_dep_gear_num]
  Demux/2 -> "shifting, out"/1, [shifting_out]
  Switch2/1 -> "gear number, out"/1, [gear_num_out]
  shifting1/1(out_1) -> [def_shifting]
  [shifting_out] -> Logical Operator1/1
  [gear_num_out] -> lock-up in this gear/1, est. engine trq and spd assuming lockup/1(new gear number)
  Demux/1 -> "gear ratio, out"/1

== system lib_transmission2/Gearbox Control/time lookup shift logic for gearbox/lookup ==
  time : Inport  Port=1  LatchInput=off
  Goto Tag Visibility : GotoTagVisibility  GotoTag=time
  gear number lookup : lib_etc/repeated signal output  t=gb_gear_number_lookup(:,1)  y=gb_gear_number_lookup(:,2)
  gear ratio lookup : Lookup  InputValues=[1:length(gb_ratio)]  OutputValues=gb_ratio
  shifting determination : Subsystem
      settings: RTWFcnNameOpts=Auto  RTWFileNameOpts=Auto
  gear ratio : Outport  Port=1  InitialOutput=0
  shifting : Outport  Port=2  InitialOutput=0
  gear number : Outport  Port=3  InitialOutput=0
  tag scope: time=scoped
  wires:
  time/1 -> [time]
  gear number lookup/1 -> gear number/1, shifting determination/1(gear number), gear ratio lookup/1
  [time] -> gear number lookup/1
  shifting determination/1(out_1) -> shifting/1
  gear ratio lookup/1 -> gear ratio/1

== system lib_transmission2/Gearbox Control/vehicle speed dependent shift logic for gearbox/speed dependent ==
  v_req_limited : Inport  Port=1  LatchInput=off
  Demux : Demux  Outputs=2  BusSelectionMode=off
  Goto Tag Visibility : GotoTagVisibility  GotoTag=v_req_limited
  Speed Dependent Shifting : Subsystem
      settings: RTWFcnNameOpts=Auto  RTWFileNameOpts=Auto
  gear ratio : Outport  Port=1  InitialOutput=0
  shifting : Outport  Port=2  InitialOutput=0
  gear number : Outport  Port=3  InitialOutput=0
  tag scope: v_req_limited=scoped
  wires:
  Speed Dependent Shifting/1(gear ratio and shifting) -> Demux/1
  Speed Dependent Shifting/2(gear number) -> gear number/1
  Demux/1 -> gear ratio/1
  Demux/2 -> shifting/1
  [v_req_limited] -> Speed Dependent Shifting/1("velocity required (limited) ")
  v_req_limited/1 -> [v_req_limited]

== system lib_transmission2/SubLibraries/loss (Nm)/Block NOTES ==
  note: Revision Notes:
  note: 09/20/02:tm modifed lower input to switch after T_loss_at_input to pass the
      | total torque input as the loss when tx_eff=0
      | 5 July 2001:mpo changing loss block to a lookup table methodology
      | 12/20/00:tm revised loss saturation block. lower limit changed
      | from 1 to 0 and upper limit changed from 100 to inf to prevent over or under penalties

== system lib_transmission2/SubLibraries/loss (Nm) old methodology/Block NOTES ==
  note: Revision Notes:
  note: 12/20/00:tm revised loss saturation block. lower limit changed
      | from 1 to 0 and upper limit changed from 100 to inf to prevent over or under penalties
